simulink model "smash_ol"  (R2016a)
settings: Solver=VariableStepAuto  StartTime=0.0  StopTime=10.0  RelTol=1e-3
values from neighbouring files (symbols this model uses):
  in =     [uav_config.mat]
  o =     [uav_config.mat]
libraries: aerolibasang x3, aerolibadyn x2, aerolib3dof2 x1, aerolibconvert2 x1, aerolibatmos2 x1
settings Model: Creator=Bilal  LastModifiedBy=Bilal

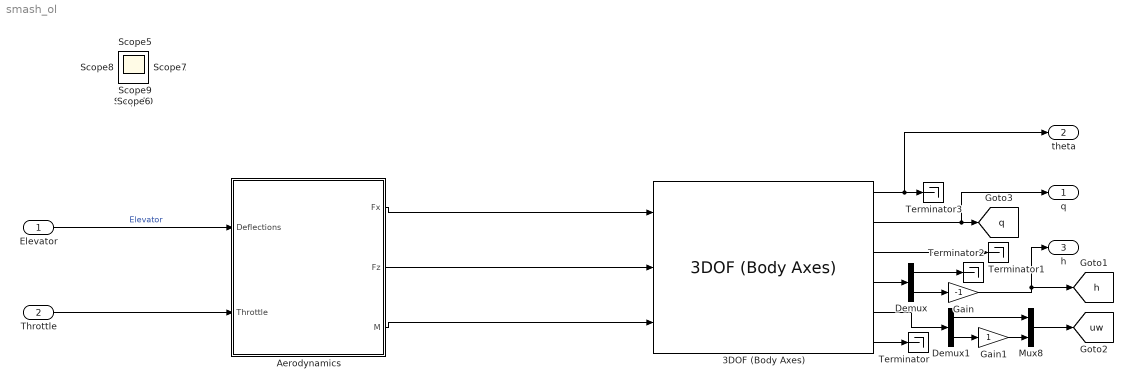
== system smash_ol ==
  Elevator : Inport
  Throttle : Inport  Port=2
  3DOF (Body Axes) : aerolib3dof2/3DOF (Body Axes)  units=Metric (MKS)  mtype=Fixed  v_ini=convvel(in.v.cr,'kts','m/s')  theta_ini=0  alpha_ini=1/pi/180  q_ini=0  pos_ini=[0 -convlength(in.alt.cr,'ft','m')]  mass=convmass(o.w0,'lbm','kg')  mass_e=0.5  mass_f=3.0  Iyy=o.Iyy*convmass(1,'slug','kg')*convlength(1,'ft','m')^2  Iyy_e=0.5  Iyy_f=3.0  g_in=Internal  g=9.81  vre_flag=on
  Aerodynamics : Subsystem
  Demux : Demux  Outputs=2
  Demux1 : Demux  Outputs=2
  Gain : Gain  Gain=-1
  Gain1 : Gain
  Mux8 : Mux  Inputs=2
  Terminator{,1..3} (4 alike) : Terminator
  q : Outport  Unit=N*m
  theta : Outport  Port=2  Unit=N*m
  h : Outport  Port=3  Unit=N*m
  Scope{,1..10} (11 alike) : Scope
  tag scope: h=global, q=global, uw=global
  wires:
  3DOF (Body Axes)/4 -> Demux/1
  Demux/2 -> Gain/1
  3DOF (Body Axes)/6 -> Terminator/1
  Gain/1 -> h/1, [h]
  Aerodynamics/1(Fx) -> 3DOF (Body Axes)/1
  Aerodynamics/2(Fz) -> 3DOF (Body Axes)/2
  Aerodynamics/3(M) -> 3DOF (Body Axes)/3
  3DOF (Body Axes)/2 -> q/1, [q]
  3DOF (Body Axes)/3 -> Terminator1/1
  Demux/1 -> Terminator2/1
  Elevator/1 -> Aerodynamics/1(Deflections)  "Elevator"
  Throttle/1 -> Aerodynamics/2(Throttle)
  3DOF (Body Axes)/5 -> Demux1/1
  Demux1/1 -> Mux8/1
  Demux1/2 -> Gain1/1
  Gain1/1 -> Mux8/2
  Mux8/1 -> [uw]
  3DOF (Body Axes)/1 -> theta/1, Terminator3/1

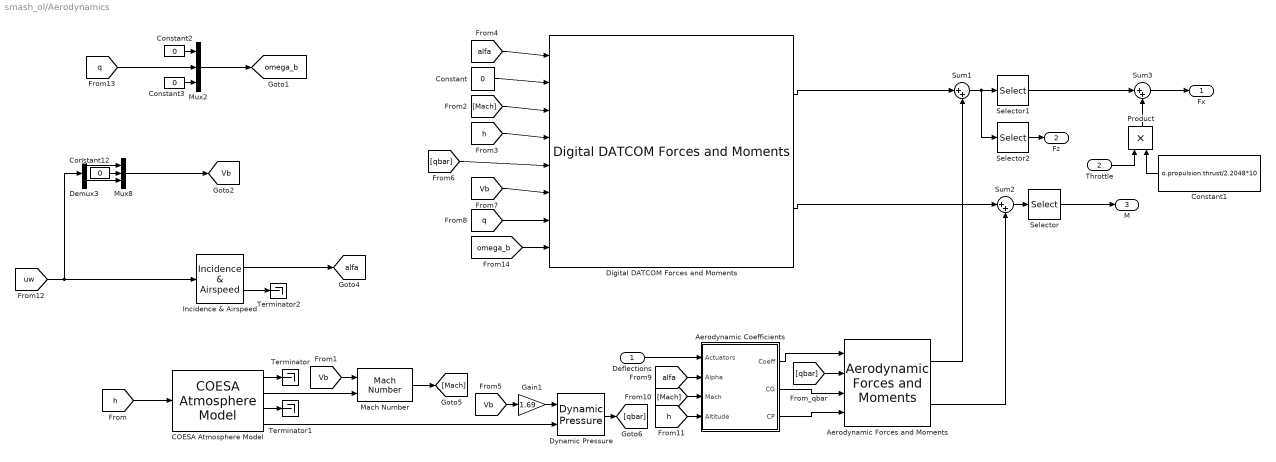
== system smash_ol/Aerodynamics ==
  Deflections : Inport
  Throttle : Inport  Port=2
  Aerodynamic Coefficients : Subsystem
  "Aerodynamic Forces and Moments " : aerolibadyn/Aerodynamic Forces and Moments   inputAxes=Body  outputForceAxes=Body  outputMomentAxes=Body  S=o.wing.S*0.3048*0.3048  b=o.wing.b*0.3048  cbar=o.wing.cmac*0.3048
  COESA Atmosphere Model : aerolibatmos2/COESA Atmosphere Model  units=Metric (MKS)  spec=1976 COESA-extended U.S. Standard Atmosphere  model=Profile  profile_var=High temperature  profile_percent=1%  profile_alt=5 km (16404 ft)  envelope_var=High temperature  envelope_percent=1%  action=Warning
  Constant{,2..3,12} (4 alike) : Constant  Value=0
  Constant1 : Constant  Value=o.propulsion.thrust/2.2048*10
  Demux3 : Demux  Outputs=2
  Digital DATCOM Forces and Moments : aerolibadyn/Digital DATCOM Forces and Moments  units=Metric (MKS)  dcase=o.aero_dc{1}  fmode=Body  buildno=0  imethod=None - flat  emethod=None - clip  rmethod=Clip to Range  action=None
  Dynamic Pressure : aerolibasang/Dynamic Pressure
  Gain1 : Gain  Gain=1.69
  Incidence & Airspeed : aerolibasang/Incidence  & Airspeed
  Mach Number : aerolibasang/Mach Number
  Mux2 : Mux  Inputs=3
  Mux8 : Mux  Inputs=3
  Product : Product
  Selector : Selector  InputPortWidth=3  IndexOptions=Index vector (dialog)  Indices=2  OutputSizes=1
  Selector1 : Selector  InputPortWidth=3  IndexOptions=Index vector (dialog)  Indices=1  OutputSizes=1
  Selector2 : Selector  InputPortWidth=3  IndexOptions=Index vector (dialog)  Indices=3  OutputSizes=1
  Sum1 : Sum  Inputs=|++
  Sum2 : Sum  Inputs=|++
  Sum3 : Sum  Inputs=|++
  Terminator : Terminator
  Terminator1 : Terminator
  Terminator2 : Terminator
  Fx : Outport  Unit=N
  Fz : Outport  Port=2  Unit=N
  M : Outport  Port=3  Unit=N*m
  tag scope: Vb=global, alfa=global, omega_b=global
  wires:
  Constant/1 -> Digital DATCOM Forces and Moments/2
  [h] -> COESA Atmosphere Model/1
  [Vb] -> Mach Number/1
  COESA Atmosphere Model/1 -> Terminator/1
  COESA Atmosphere Model/3 -> Terminator1/1
  Mach Number/1 -> [Mach]
  [Mach] -> Digital DATCOM Forces and Moments/3
  [h] -> Digital DATCOM Forces and Moments/4
  [alfa] -> Digital DATCOM Forces and Moments/1
  COESA Atmosphere Model/4 -> Dynamic Pressure/2
  Dynamic Pressure/1 -> [qbar]
  [Vb] -> Digital DATCOM Forces and Moments/6
  Aerodynamic Coefficients/1(Coeff) -> "Aerodynamic Forces and Moments "/1
  "Aerodynamic Forces and Moments "/1 -> Sum1/2
  "Aerodynamic Forces and Moments "/2 -> Sum2/2
  Aerodynamic Coefficients/2(CG) -> "Aerodynamic Forces and Moments "/3
  Aerodynamic Coefficients/3(CP) -> "Aerodynamic Forces and Moments "/4
  [qbar] -> "Aerodynamic Forces and Moments "/2
  Digital DATCOM Forces and Moments/1 -> Sum1/1
  Digital DATCOM Forces and Moments/2 -> Sum2/1
  Sum2/1 -> Selector/1
  [alfa] -> Aerodynamic Coefficients/2(Alpha)
  [Mach] -> Aerodynamic Coefficients/3(Mach)
  [h] -> Aerodynamic Coefficients/4(Altitude)
  Selector/1 -> M/1
  Selector2/1 -> Fz/1
  Sum1/1 -> Selector2/1, Selector1/1
  Deflections/1 -> Aerodynamic Coefficients/1(Actuators)
  Incidence & Airspeed/2 -> Terminator2/1
  COESA Atmosphere Model/2 -> Mach Number/2
  Demux3/2 -> Mux8/3
  Constant12/1 -> Mux8/2
  Demux3/1 -> Mux8/1
  [uw] -> Incidence & Airspeed/1, Demux3/1
  Mux8/1 -> [Vb]
  Selector1/1 -> Sum3/1
  Sum3/1 -> Fx/1
  [q] -> Mux2/2
  Constant2/1 -> Mux2/1
  Constant3/1 -> Mux2/3
  Mux2/1 -> [omega_b]
  [qbar] -> Digital DATCOM Forces and Moments/5
  [Vb] -> Gain1/1
  Gain1/1 -> Dynamic Pressure/1
  Constant1/1 -> Product/2
  Throttle/1 -> Product/1
  Product/1 -> Sum3/2
  Incidence & Airspeed/1 -> [alfa]
  [omega_b] -> Digital DATCOM Forces and Moments/8
  [q] -> Digital DATCOM Forces and Moments/7

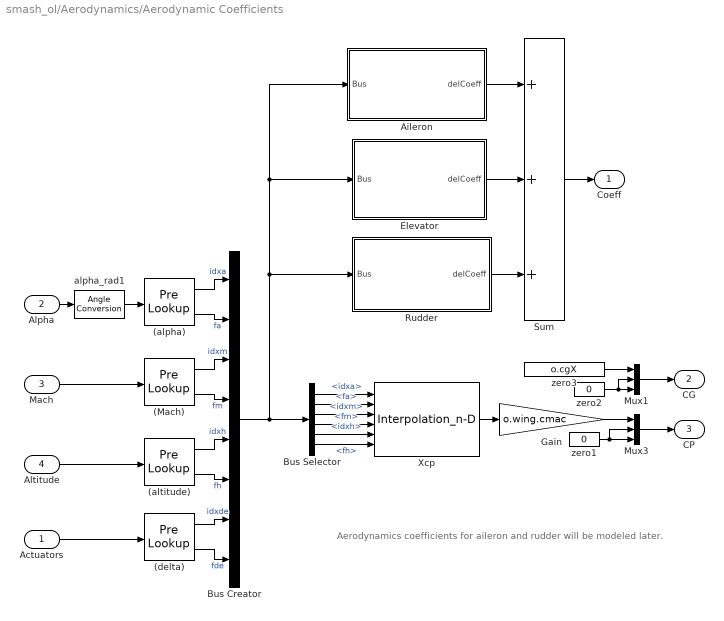
== system smash_ol/Aerodynamics/Aerodynamic Coefficients ==
  note: Aerodynamics coefficients for aileron and rudder will be modeled later.
  Actuators : Inport
  Alpha : Inport  Port=2
  Mach : Inport  Port=3
  Altitude : Inport  Port=4
  (Mach) : PreLookup  BreakpointsData=o.aero_dc{1}.mach  BeginIndexSearchUsingPreviousIndexResult=on  ExtrapMethod=Linear  IndexDataTypeStr=int32  FractionDataTypeStr=double
  (alpha) : PreLookup  BreakpointsData=o.aero_dc{1}.alpha  BeginIndexSearchUsingPreviousIndexResult=on  ExtrapMethod=Linear  IndexDataTypeStr=int32  FractionDataTypeStr=double
  (altitude) : PreLookup  BreakpointsData=o.aero_dc{1}.alt  BeginIndexSearchUsingPreviousIndexResult=on  ExtrapMethod=Linear  IndexDataTypeStr=int32  FractionDataTypeStr=double
  (delta) : PreLookup  BreakpointsData=o.aero_dc{1}.delta  BeginIndexSearchUsingPreviousIndexResult=on  ExtrapMethod=Linear  IndexDataTypeStr=int32  FractionDataTypeStr=double
  Aileron : Subsystem
  Bus Creator : BusCreator  Inputs=8
  Bus Selector : BusSelector  OutputSignals=idxa,fa,idxm,fm,idxh,fh
  Elevator : Subsystem
  Gain : Gain  Gain=o.wing.cmac
  Mux1 : Mux  Inputs=3
  Mux3 : Mux  Inputs=3
  Rudder : Subsystem
  Sum : Sum  Inputs=3  SaturateOnIntegerOverflow=on  InputSameDT=on  OutDataTypeStr=Inherit: Same as first input
  Xcp : Interpolation_n-D  NumberOfTableDimensions=3  Table="permute(o.aero_dc{1}.xcp,[1  2  3])"  OutDataTypeStr=double
      settings: InputPortMap=u0,u1,u2,u3,u4,u5
  alpha_rad1 : aerolibconvert2/Angle Conversion  IU=rad  OU=deg
  zero1 : Constant  Value=0
  zero2 : Constant  Value=0
  zero3 : Constant  Value=o.cgX
  Coeff : Outport  InitialOutput=0
  CG : Outport  Port=2  PortDimensions=3  InitialOutput=0
  CP : Outport  Port=3  PortDimensions=3  InitialOutput=0
  wires:
  Sum/1 -> Coeff/1
  Mux1/1 -> CG/1
  Mux3/1 -> CP/1
  Xcp/1 -> Gain/1
  zero1/1 -> Mux3/2, Mux3/3
  Gain/1 -> Mux3/1
  (alpha)/2 -> Bus Creator/2  "fa"
  (Mach)/2 -> Bus Creator/4  "fm"
  (altitude)/2 -> Bus Creator/6  "fh"
  (altitude)/1 -> Bus Creator/5  "idxh"
  (Mach)/1 -> Bus Creator/3  "idxm"
  (alpha)/1 -> Bus Creator/1  "idxa"
  Bus Selector/1 -> Xcp/1  "<idxa>"
  Bus Selector/2 -> Xcp/2  "<fa>"
  Bus Selector/3 -> Xcp/3  "<idxm>"
  Bus Selector/4 -> Xcp/4  "<fm>"
  Bus Selector/5 -> Xcp/5  "<idxh>"
  Bus Selector/6 -> Xcp/6  "<fh>"
  Bus Creator/1 -> Bus Selector/1, Elevator/1(Bus), Aileron/1(Bus), Rudder/1(Bus)
  Mach/1 -> (Mach)/1
  Altitude/1 -> (altitude)/1
  Alpha/1 -> alpha_rad1/1
  alpha_rad1/1 -> (alpha)/1
  Aileron/1(delCoeff) -> Sum/1
  Elevator/1(delCoeff) -> Sum/2
  Rudder/1(delCoeff) -> Sum/3
  (delta)/1 -> Bus Creator/7  "idxde"
  (delta)/2 -> Bus Creator/8  "fde"
  Actuators/1 -> (delta)/1
  zero2/1 -> Mux1/3, Mux1/2
  zero3/1 -> Mux1/1

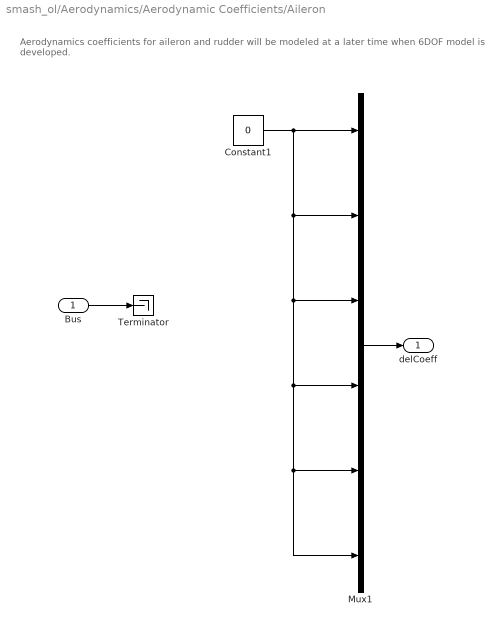
== system smash_ol/Aerodynamics/Aerodynamic Coefficients/Aileron ==
  note: Aerodynamics coefficients for aileron and rudder will be modeled at a later time when 6DOF model is developed.
  Bus : Inport
  Constant1 : Constant  Value=0
  Mux1 : Mux  Inputs=6
  Terminator : Terminator
  delCoeff : Outport
  wires:
  Mux1/1 -> delCoeff/1
  Constant1/1 -> Mux1/1, Mux1/2, Mux1/3, Mux1/4, Mux1/5, Mux1/6
  Bus/1 -> Terminator/1

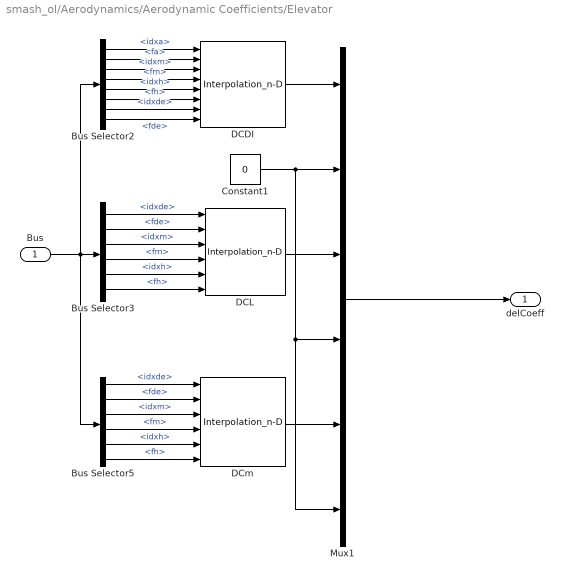
== system smash_ol/Aerodynamics/Aerodynamic Coefficients/Elevator ==
  Bus : Inport
  Bus Selector2 : BusSelector  OutputSignals=idxa,fa,idxm,fm,idxh,fh,idxde,fde
  Bus Selector3 : BusSelector  OutputSignals=idxde,fde,idxm,fm,idxh,fh
  Bus Selector5 : BusSelector  OutputSignals=idxde,fde,idxm,fm,idxh,fh
  Constant1 : Constant  Value=0
  DCDI : Interpolation_n-D  NumberOfTableDimensions=4  Table=permute(o.aero_dc{1}.dcdi_sym,[1 3 4 2 ])  RemoveProtectionIndex=on
      settings: InputPortMap=u0,u1,u2,u3,u4,u5,u6,u7
  DCL : Interpolation_n-D  NumberOfTableDimensions=3  Table="permute(o.aero_dc{1}.dcl_sym,[1  2  3])"  RemoveProtectionIndex=on
      settings: InputPortMap=u0,u1,u2,u3,u4,u5
  DCm : Interpolation_n-D  NumberOfTableDimensions=3  Table="permute(o.aero_dc{1}.dcm_sym,[1  2  3])"  RemoveProtectionIndex=on
      settings: InputPortMap=u0,u1,u2,u3,u4,u5
  Mux1 : Mux  Inputs=6
  delCoeff : Outport
  wires:
  Mux1/1 -> delCoeff/1
  Bus/1 -> Bus Selector2/1, Bus Selector3/1, Bus Selector5/1
  DCDI/1 -> Mux1/1
  DCL/1 -> Mux1/3
  DCm/1 -> Mux1/5
  Constant1/1 -> Mux1/2, Mux1/4, Mux1/6
  Bus Selector2/1 -> DCDI/1  "<idxa>"
  Bus Selector2/2 -> DCDI/2  "<fa>"
  Bus Selector3/1 -> DCL/1  "<idxde>"
  Bus Selector3/2 -> DCL/2  "<fde>"
  Bus Selector5/1 -> DCm/1  "<idxde>"
  Bus Selector5/2 -> DCm/2  "<fde>"
  Bus Selector2/3 -> DCDI/3  "<idxm>"
  Bus Selector2/4 -> DCDI/4  "<fm>"
  Bus Selector2/5 -> DCDI/5  "<idxh>"
  Bus Selector2/6 -> DCDI/6  "<fh>"
  Bus Selector2/7 -> DCDI/7  "<idxde>"
  Bus Selector2/8 -> DCDI/8  "<fde>"
  Bus Selector3/3 -> DCL/3  "<idxm>"
  Bus Selector3/4 -> DCL/4  "<fm>"
  Bus Selector3/5 -> DCL/5  "<idxh>"
  Bus Selector3/6 -> DCL/6  "<fh>"
  Bus Selector5/3 -> DCm/3  "<idxm>"
  Bus Selector5/4 -> DCm/4  "<fm>"
  Bus Selector5/5 -> DCm/5  "<idxh>"
  Bus Selector5/6 -> DCm/6  "<fh>"

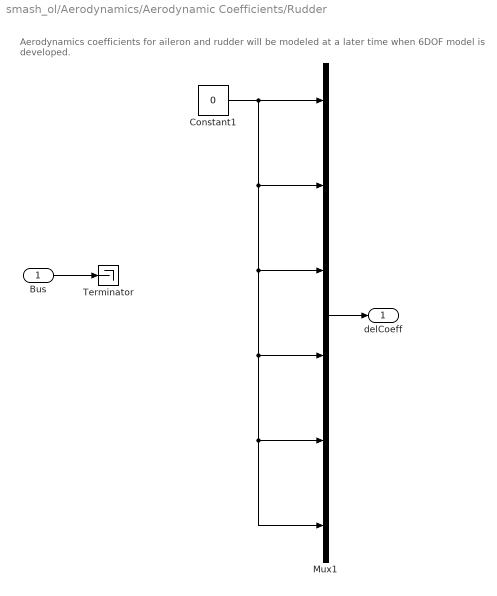
== system smash_ol/Aerodynamics/Aerodynamic Coefficients/Rudder ==
  note: Aerodynamics coefficients for aileron and rudder will be modeled at a later time when 6DOF model is developed.
  Bus : Inport
  Constant1 : Constant  Value=0
  Mux1 : Mux  Inputs=6
  Terminator : Terminator
  delCoeff : Outport
  wires:
  Mux1/1 -> delCoeff/1
  Constant1/1 -> Mux1/6, Mux1/5, Mux1/4, Mux1/3, Mux1/2, Mux1/1
  Bus/1 -> Terminator/1
